simulink model "TestMyFun3te"  (R2013b)
settings: Solver=ode45  StartTime=0.0  StopTime=1  RelTol=1e-3
libraries: simulink x1
Description:
  | output Te, to check
settings Model: Creator=Think79  LastModifiedBy=Think79

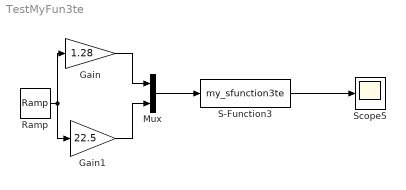
== system TestMyFun3te ==
  Gain : Gain  Gain=1.28
  Gain1 : Gain  Gain=22.5
  Mux : Mux  Inputs=2
  Ramp : simulink/Sources/Ramp  slope=1  start=0  X0=0
  S-Function3 : S-Function  FunctionName=my_sfunction3te  EnableBusSupport=off
  Scope5 : Scope
      settings: YMin=-0.25  YMax=2
  wires:
  Mux/1 -> S-Function3/1
  Gain/1 -> Mux/1
  S-Function3/1 -> Scope5/1
  Ramp/1 -> Gain/1, Gain1/1
  Gain1/1 -> Mux/2
